simulink model "Actuators"  (Simulink 8.4)
settings: Solver=ode45  StartTime=0.0  StopTime=10.0  RelTol=1e-3
undefined symbols (not defined in the file): Ais_flgAirInjReacPumpOverride, Ais_stAirInjReacPumpMan, Apv_facAirPumpRateMan, Apv_factor, Apv_flgAirPumpRateOverride, Apv_tiPeriod_C, CDRV_E_OK_, Cov_facChOverVlvRateMan, Cov_factor, Cov_flgChOverVlvRateOverride, Cov_tiPeriod_C, Doh_OutputDiagnosisOverride, Fps_flgFuelPumpOverride, Fps_stFuelPumpMan, Icc_degIgnMan, Icc_flgIgnAngleOverride, Icc_flgIgnCutoffMan, Icc_flgIgnCutoffOverride, Icc_nrFollowUpSparks, Icc_tiDwell, Icc_tiDwellFollowUpSparks, Icc_tiOffFollowUpSparks, Ics_flgIntercoolerOverride, Ics_stIntercoolerMan, Ivc_degInjAbort, Ivc_degIntakeClose, Ivc_degOffsetInjEndSimultanInj, Ivc_flgBattDelayOverride, Ivc_flgDiagEntryCondFulfilled, Ivc_flgEndOfStartCond, Ivc_flgInjCutoff, Ivc_flgInjCutoffOverride, Ivc_flgInjTimeOverride, Ivc_flgOverrunCutoff, Ivc_flgPostInjCond, Ivc_tiBattDelayMan, Ivc_tiInjEff, Ivc_tiInjMan, Ivc_tiMinThresDeltaEffInjPeriod, Ivc_weea0, Ivc_weea1, Ivc_weea2, Lo_, Mrs_flgMainRelaisOverride, Mrs_stMainRelaisMan, Normal, OK, OpenCircuit, OverTemp, ShortToBatt, ShortToBattNEG, ShortToGnd, ShortToGndNEG, ShortToGndPOS, Str_flgStarterOverride, Str_stStarterMan, Tvc_facDutycyclePIDLimitMax, Tvc_facDutycyclePIDLimitMin, Tvc_facDutycyclePilotControlNeg, Tvc_facDutycyclePilotControlPos ... (+20)
libraries: simulink x9
(part 1 of 3)
settings Model: Creator=YAL9FE  LastModifiedBy=ric9fe
settings DebuggingCC: FcnCallInpInsideContextMsg=EnableAllAsWarning

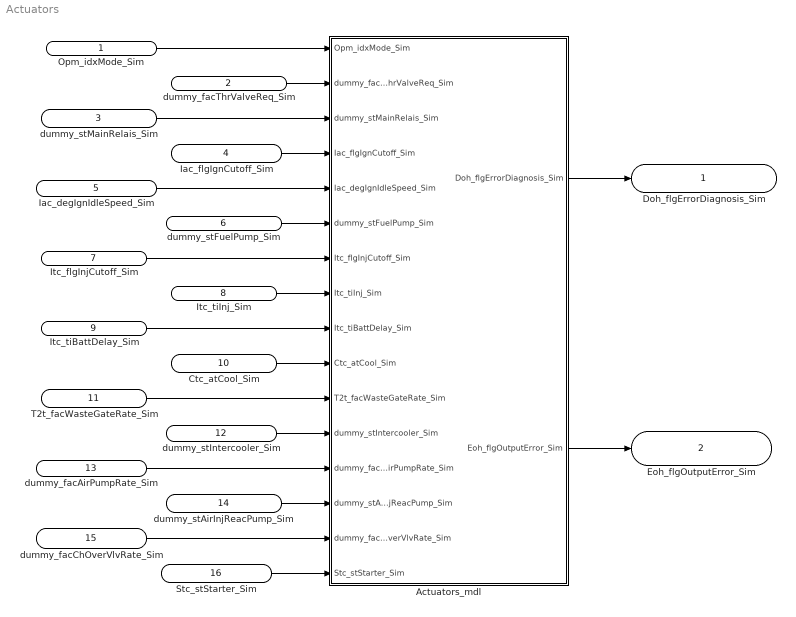
== system Actuators ==
  Opm_idxMode_Sim : Inport
  dummy_facThrValveReq_Sim : Inport  Port=2
  dummy_stMainRelais_Sim : Inport  Port=3
  Iac_flgIgnCutoff_Sim : Inport  Port=4
  Iac_degIgnIdleSpeed_Sim : Inport  Port=5
  dummy_stFuelPump_Sim : Inport  Port=6
  Itc_flgInjCutoff_Sim : Inport  Port=7
  Itc_tiInj_Sim : Inport  Port=8
  Itc_tiBattDelay_Sim : Inport  Port=9
  Ctc_atCool_Sim : Inport  Port=10
  T2t_facWasteGateRate_Sim : Inport  Port=11
  dummy_stIntercooler_Sim : Inport  Port=12
  dummy_facAirPumpRate_Sim : Inport  Port=13
  dummy_stAirInjReacPump_Sim : Inport  Port=14
  dummy_facChOverVlvRate_Sim : Inport  Port=15
  Stc_stStarter_Sim : Inport  Port=16
  Actuators_mdl : Subsystem
  Doh_flgErrorDiagnosis_Sim : Outport
  Eoh_flgOutputError_Sim : Outport  Port=2
  wires:
  Opm_idxMode_Sim/1 -> Actuators_mdl/1(Opm_idxMode_Sim)
  dummy_facThrValveReq_Sim/1 -> Actuators_mdl/2(dummy_facThrValveReq_Sim)
  dummy_stMainRelais_Sim/1 -> Actuators_mdl/3(dummy_stMainRelais_Sim)
  Iac_flgIgnCutoff_Sim/1 -> Actuators_mdl/4(Iac_flgIgnCutoff_Sim)
  Iac_degIgnIdleSpeed_Sim/1 -> Actuators_mdl/5(Iac_degIgnIdleSpeed_Sim)
  dummy_stFuelPump_Sim/1 -> Actuators_mdl/6(dummy_stFuelPump_Sim)
  Itc_flgInjCutoff_Sim/1 -> Actuators_mdl/7(Itc_flgInjCutoff_Sim)
  Itc_tiInj_Sim/1 -> Actuators_mdl/8(Itc_tiInj_Sim)
  Itc_tiBattDelay_Sim/1 -> Actuators_mdl/9(Itc_tiBattDelay_Sim)
  Ctc_atCool_Sim/1 -> Actuators_mdl/10(Ctc_atCool_Sim)
  T2t_facWasteGateRate_Sim/1 -> Actuators_mdl/11(T2t_facWasteGateRate_Sim)
  dummy_stIntercooler_Sim/1 -> Actuators_mdl/12(dummy_stIntercooler_Sim)
  dummy_facAirPumpRate_Sim/1 -> Actuators_mdl/13(dummy_facAirPumpRate_Sim)
  dummy_stAirInjReacPump_Sim/1 -> Actuators_mdl/14(dummy_stAirInjReacPump_Sim)
  dummy_facChOverVlvRate_Sim/1 -> Actuators_mdl/15(dummy_facChOverVlvRate_Sim)
  Stc_stStarter_Sim/1 -> Actuators_mdl/16(Stc_stStarter_Sim)
  Actuators_mdl/1(Doh_flgErrorDiagnosis_Sim) -> Doh_flgErrorDiagnosis_Sim/1
  Actuators_mdl/2(Eoh_flgOutputError_Sim) -> Eoh_flgOutputError_Sim/1

== system Actuators/Actuators_mdl ==
  Opm_idxMode_Sim : Inport
  dummy_facThrValveReq_Sim : Inport  Port=2
  dummy_stMainRelais_Sim : Inport  Port=3
  Iac_flgIgnCutoff_Sim : Inport  Port=4
  Iac_degIgnIdleSpeed_Sim : Inport  Port=5
  dummy_stFuelPump_Sim : Inport  Port=6
  Itc_flgInjCutoff_Sim : Inport  Port=7
  Itc_tiInj_Sim : Inport  Port=8
  Itc_tiBattDelay_Sim : Inport  Port=9
  Ctc_atCool_Sim : Inport  Port=10
  T2t_facWasteGateRate_Sim : Inport  Port=11
  dummy_stIntercooler_Sim : Inport  Port=12
  dummy_facAirPumpRate_Sim : Inport  Port=13
  dummy_stAirInjReacPump_Sim : Inport  Port=14
  dummy_facChOverVlvRate_Sim : Inport  Port=15
  Stc_stStarter_Sim : Inport  Port=16
  Ais : Subsystem  mask(Actuators){}
      mask help: AirInjectionReactorPump
      mask Display:
      | image(imread('AirInjectionReactorPump.jpg'))
      | port_label('input',1,'Opm_idxMode_Sim')
      | port_label('input',2,'dummy_stAirInjReacPump_Sim')
      | port_label('output',1,'Ais_stDiagnosis')
      | port_label('output',2,'Ais_flgError')
  Apv : Subsystem  mask(Actuators){}
      mask help: AirPumpValve
      mask Display:
      | image(imread('AirPumpValve.jpg'))
      | port_label('input',1,'Opm_idxMode_Sim')
      | port_label('input',2,'dummy_facAirPumpRate_Sim')
      | port_label('output',1,'Apv_stDiagnosis')
      | port_label('output',2,'Apv_flgError')
  Cov : Subsystem  mask(Actuators){}
      mask help: ChangeOverValve
      mask Display:
      | image(imread('ChangeOverValve.jpg'))
      | port_label('input',1,'Opm_idxMode_Sim')
      | port_label('input',2,'dummy_facChOverVlvRate_Sim')
      | port_label('output',1,'Cov_stDiagnosis')
      | port_label('output',2,'Cov_flgError')
  Doh : Subsystem  AncestorBlock=M160_lib/Functions/Eih  mask(Functions){}
      mask help: DiagnosisOutput
      mask Display:
      | image(imread('DiagnosisOutput.jpg'))
      | port_label('input',1,'Tvc_stDiagnosis')
      | port_label('input',2,'Mrs_stDiagnosis')
      | port_label('input',3,'Fps_stDiagnosis')
      | port_label('input',4,'Wcs_stDiagnosis')
      | port_label('input',5,'Wgc_stDiagnosis')
      | port_label('input',6,'Ics_stDiagnosis')
      | port_label('input',7,'Apv_stDiagnosis')
      | port_label('input',8,'Ais_stDiagnosis')
      | port_label('input',9,'Cov_stDiagnosis')
      | port_label('input',10,'Str_stDiagnosis')
      | port_label('output',1,'Doh_flgErrorDiagnosis_Sim')
  Eoh : Subsystem  AncestorBlock=M160_lib/Functions/Eih  mask(Functions){}
      mask help: ErrorOutput
      mask Display:
      | image(imread('ErrorOutput.jpg'))
      | port_label('input',1,'Tvc_flgError')
      | port_label('input',2,'Mrs_flgError')
      | port_label('input',3,'Icc_flgError')
      | port_label('input',4,'Fps_flgError')
      | port_label('input',5,'Ivc_flgError')
      | port_label('input',6,'Wcs_flgError')
      | port_label('input',7,'Wgc_flgError')
      | port_label('input',8,'Ics_flgError')
      | port_label('input',9,'Apv_flgError')
      | port_label('input',10,'Ais_flgError')
      | port_label('input',11,'Cov_flgError')
      | port_label('input',12,'Str_flgError')
      | port_label('output',1,'Eoh_flgOutputError_Sim')
  Fps : Subsystem  mask(Actuators){}
      mask help: FuelPump
      mask Display:
      | image(imread('FuelPump.jpg'))
      | port_label('input',1,'Opm_idxMode_Sim')
      | port_label('input',2,'dummy_stFuelPump_Sim')
      | port_label('output',1,'Fps_stDiagnosis')
      | port_label('output',2,'Fps_flgError')
  Icc : Subsystem  mask(Actuators){}
      mask help: IgnitionCoil
      mask Display:
      | image(imread('IgnitionCoil.jpg'))
      | port_label('input',1,'Opm_idxMode_Sim')
      | port_label('input',2,'Iac_flgIgnCutoff_Sim')
      | port_label('input',3,'Iac_degIgnIdleSpeed_Sim')
      | port_label('output',1,'Icc_flgError')
  Ics : Subsystem  mask(Actuators){}
      mask help: Intercooler
      mask Display:
      | image(imread('Intercooler.jpg'))
      | port_label('input',1,'Opm_idxMode_Sim')
      | port_label('input',2,'dummy_stIntercooler_Sim')
      | port_label('output',1,'Ics_stDiagnosis')
      | port_label('output',2,'Ics_flgError')
  Ivc : Subsystem  mask(Actuators){}
      mask help: InjectionValve
      mask Display:
      | image(imread('InjectionValve.jpg'))
      | port_label('input',1,'Opm_idxMode_Sim')
      | port_label('input',2,'Itc_flgInjCutoff_Sim')
      | port_label('input',3,'Itc_tiInj_Sim')
      | port_label('input',4,'Itc_tiBattDelay_Sim')
      | port_label('output',1,'Ivc_flgError')
  Mrs : Subsystem  mask(Actuators){}
      mask help: MainRelais
      mask Display:
      | image(imread('MainRelais.jpg'))
      | port_label('input',1,'Opm_idxMode_Sim')
      | port_label('input',2,'dummy_stMainRelais_Sim')
      | port_label('output',1,'Mrs_stDiagnosis')
      | port_label('output',2,'Mrs_flgError')
  Str : Subsystem  mask(Actuators){}
      mask help: Starter
      mask Display:
      | image(imread('Starter.jpg'))
      | port_label('input',1,'Opm_idxMode_Sim')
      | port_label('input',2,'Stc_stStarter_Sim')
      | port_label('output',1,'Str_stDiagnosis')
      | port_label('output',2,'Str_flgError')
  Tvc : Subsystem  mask(Actuators){}
      mask help: ThrottleValve
      mask Display:
      | image(imread('ThrottleValve.jpg'))
      | port_label('input',1,'Opm_idxMode_Sim')
      | port_label('input',2,'dummy_facThrValveReq_Sim')
      | port_label('output',1,'Tvc_stDiagnosis')
      | port_label('output',2,'Tvc_flgError')
  Wcs : Subsystem  mask(Actuators){}
      mask help: WaterCooler
      mask Display:
      | image(imread('WaterCooler.jpg'))
      | port_label('input',1,'Opm_idxMode_Sim')
      | port_label('input',2,'Ctc_atCool_Sim')
      | port_label('output',1,'Wcs_stDiagnosis')
      | port_label('output',2,'Wcs_flgError')
  Wgc : Subsystem  mask(Actuators){}
      mask help: WasteGate
      mask Display:
      | image(imread('WasteGate.jpg'))
      | port_label('input',1,'Opm_idxMode_Sim')
      | port_label('input',2,'T2t_facWasteGateRate_Sim')
      | port_label('output',1,'Wgc_stDiagnosis')
      | port_label('output',2,'Wgc_flgError')
  Doh_flgErrorDiagnosis_Sim : Outport
  Eoh_flgOutputError_Sim : Outport  Port=2
  wires:
  Icc/1(Icc_flgError) -> Eoh/3(Icc_flgError)
  Mrs/2(Mrs_flgError) -> Eoh/2(Mrs_flgError)
  Tvc/2(Tvc_flgError) -> Eoh/1(Tvc_flgError)
  Eoh/1(Eoh_flgOutputError_Sim) -> Eoh_flgOutputError_Sim/1
  Stc_stStarter_Sim/1 -> Str/2(Stc_stStarter_Sim)
  Str/1(Str_stDiagnosis) -> Doh/10(Str_stDiagnosis)
  dummy_facChOverVlvRate_Sim/1 -> Cov/2(dummy_facChOverVlvRate_Sim)
  Cov/1(Cov_stDiagnosis) -> Doh/9(Cov_stDiagnosis)
  dummy_stAirInjReacPump_Sim/1 -> Ais/2(dummy_stAirInjReacPump_Sim)
  dummy_facAirPumpRate_Sim/1 -> Apv/2(dummy_facAirPumpRate_Sim)
  Fps/2(Fps_flgError) -> Eoh/4(Fps_flgError)
  Ivc/1(Ivc_flgError) -> Eoh/5(Ivc_flgError)
  Wcs/2(Wcs_flgError) -> Eoh/6(Wcs_flgError)
  Wgc/2(Wgc_flgError) -> Eoh/7(Wgc_flgError)
  Ics/2(Ics_flgError) -> Eoh/8(Ics_flgError)
  Apv/2(Apv_flgError) -> Eoh/9(Apv_flgError)
  Ais/2(Ais_flgError) -> Eoh/10(Ais_flgError)
  Cov/2(Cov_flgError) -> Eoh/11(Cov_flgError)
  Str/2(Str_flgError) -> Eoh/12(Str_flgError)
  Doh/1(Doh_flgErrorDiagnosis_Sim) -> Doh_flgErrorDiagnosis_Sim/1
  Opm_idxMode_Sim/1 -> Tvc/1(Opm_idxMode_Sim), Mrs/1(Opm_idxMode_Sim), Icc/1(Opm_idxMode_Sim), Fps/1(Opm_idxMode_Sim), Ivc/1(Opm_idxMode_Sim), Wcs/1(Opm_idxMode_Sim), Wgc/1(Opm_idxMode_Sim), Apv/1(Opm_idxMode_Sim), Ais/1(Opm_idxMode_Sim), Cov/1(Opm_idxMode_Sim), Str/1(Opm_idxMode_Sim), Ics/1(Opm_idxMode_Sim)
  Ais/1(Ais_stDiagnosis) -> Doh/8(Ais_stDiagnosis)
  Apv/1(Apv_stDiagnosis) -> Doh/7(Apv_stDiagnosis)
  dummy_stIntercooler_Sim/1 -> Ics/2(dummy_stIntercooler_Sim)
  Ics/1(Ics_stDiagnosis) -> Doh/6(Ics_stDiagnosis)
  T2t_facWasteGateRate_Sim/1 -> Wgc/2(T2t_facWasteGateRate_Sim)
  Wgc/1(Wgc_stDiagnosis) -> Doh/5(Wgc_stDiagnosis)
  Ctc_atCool_Sim/1 -> Wcs/2(Ctc_atCool_Sim)
  Wcs/1(Wcs_stDiagnosis) -> Doh/4(Wcs_stDiagnosis)
  Itc_tiBattDelay_Sim/1 -> Ivc/4(Itc_tiBattDelay_Sim)
  Itc_tiInj_Sim/1 -> Ivc/3(Itc_tiInj_Sim)
  Itc_flgInjCutoff_Sim/1 -> Ivc/2(Itc_flgInjCutoff_Sim)
  dummy_stFuelPump_Sim/1 -> Fps/2(dummy_stFuelPump_Sim)
  Fps/1(Fps_stDiagnosis) -> Doh/3(Fps_stDiagnosis)
  Iac_degIgnIdleSpeed_Sim/1 -> Icc/3(Iac_degIgnIdleSpeed_Sim)
  Iac_flgIgnCutoff_Sim/1 -> Icc/2(Iac_flgIgnCutoff_Sim)
  dummy_stMainRelais_Sim/1 -> Mrs/2(dummy_stMainRelais_Sim)
  Mrs/1(Mrs_stDiagnosis) -> Doh/2(Mrs_stDiagnosis)
  Tvc/1(Tvc_stDiagnosis) -> Doh/1(Tvc_stDiagnosis)
  dummy_facThrValveReq_Sim/1 -> Tvc/2(dummy_facThrValveReq_Sim)
  ? -> Cov/Trigger

== system Actuators/Actuators_mdl/Ais ==
  Opm_idxMode_Sim : Inport
  dummy_stAirInjReacPump_Sim : Inport  Port=2
  function : TriggerPort  TriggerType=function-call
  Constant1 : Constant  Value=Ais_flgAirInjReacPumpOverride
  Constant2 : Constant  Value=Ais_stAirInjReacPumpMan
  Constant5 : Constant  Value=Normal
  Constant6 : Constant  Value=0  OutDataTypeStr=boolean
  G1_DigOut_Ctrl : Subsystem  AncestorBlock=ehooks_medc17flex_G1_lib/Library Blocks/Basic_IO/Outputs/G1_DigOut_Ctrl  mask{ChannelName=O_S_RL30}
      mask prompts: ChannelName "Channel name"
      mask init:
      | ehooks_medc17flex_devlib_io_block('mask_init');
      settings: AttributesFormatString=Channel name: '%<ChannelName>'
      mask TypeOptions ChannelName: <empty> | O_S_MRLY | O_S_RL09 | O_S_RL14 | O_S_RL29 | O_S_RL30 | O_S_RL31 | O_S_RL33 | O_S_RL34 | O_S_RL35 | O_S_RL41 | O_S_RL43
      mask Display: image(imread('Output_Digital.jpg'))
  G1_DigOut_GetError : Subsystem  AncestorBlock=ehooks_medc17flex_G1_lib/Library Blocks/Basic_IO/Outputs/G1_DigOut_GetError  mask{ChannelName=O_S_RL30}
      mask prompts: ChannelName "Channel name"
      mask init:
      | ehooks_medc17flex_devlib_io_block('mask_init');
      settings: AttributesFormatString=Channel name: '%<ChannelName>'
      mask TypeOptions ChannelName: <empty> | O_S_MRLY | O_S_RL09 | O_S_RL14 | O_S_RL29 | O_S_RL30 | O_S_RL31 | O_S_RL33 | O_S_RL34 | O_S_RL35 | O_S_RL41 | O_S_RL43
      mask Display: image(imread('Output_Digital_Diagnosis.jpg'))
  Logical Operator1 : Logic  Operator=NOT  AllPortsSameDT=off  OutDataTypeStr=boolean
  Logical Operator2 : Logic  Operator=NOT  AllPortsSameDT=off  OutDataTypeStr=boolean
  Relational Operator : RelationalOperator  Operator===  OutDataTypeStr=boolean
  Switch1 : Switch  Threshold=1
  Switch2 : Switch  Threshold=1
  Ais_stDiagnosis : Outport
  Ais_flgError : Outport  Port=2
  wires:
  G1_DigOut_Ctrl/1(status) -> Logical Operator1/1
  Logical Operator2/1 -> G1_DigOut_Ctrl/1(state)
  Switch2/1 -> Logical Operator2/1  "Ais_stAirInjReacPump"
  G1_DigOut_GetError/1(status) -> Ais_stDiagnosis/1  "Ais_stDiagnosis"
  Logical Operator1/1 -> Ais_flgError/1  "Ais_flgError"
  Constant1/1 -> Switch1/2
  Constant2/1 -> Switch1/1
  dummy_stAirInjReacPump_Sim/1 -> Switch1/3
  Switch1/1 -> Switch2/1
  Opm_idxMode_Sim/1 -> Relational Operator/1
  Constant5/1 -> Relational Operator/2
  Relational Operator/1 -> Switch2/2
  Constant6/1 -> Switch2/3

== system Actuators/Actuators_mdl/Apv ==
  Opm_idxMode_Sim : Inport
  dummy_facAirPumpRate_Sim : Inport  Port=2
  function : TriggerPort  TriggerType=function-call
  Constant1 : Constant  Value=Apv_flgAirPumpRateOverride
  Constant2 : Constant  Value=Apv_facAirPumpRateMan
  Constant3 : Constant  Value=10000  OutDataTypeStr=single
  Constant4 : Constant  Value=Apv_factor
  Constant5 : Constant  Value=Normal
  Constant6 : Constant  Value=0.05  OutDataTypeStr=single
  Constant7 : Constant  Value=Apv_tiPeriod_C
  Constant9 : Constant  Value=Lo_
  G1_PWM_Output_Ctrl : Subsystem  AncestorBlock=ehooks_medc17flex_G1_lib/Library Blocks/Basic_IO/Outputs/G1_PWM_Output_Ctrl  mask{ChannelName=O_T_RL13}
      mask prompts: ChannelName "Channel name"
      mask init:
      | ehooks_medc17flex_devlib_io_block('mask_init');
      settings: AttributesFormatString=Channel name: '%<ChannelName>'
      mask TypeOptions ChannelName: <empty> | O_T_RL10 | O_T_RL13 | O_T_RL19 | O_T_RL20 | O_T_RL22 | O_T_RL23 | O_T_RL25 | O_T_RL26 | O_T_RL27 | O_T_RL28 | O_T_RL38 | O_T_RL39 | O_T_RL40 | O_T_RL42 | O_T_RL44 | O_T_RL45 | O_T_RL46 | O_T_RL47 | O_T_RL48 | O_T_RL49 | O_T_RL50 | O_T_RH02
      mask Display: image(imread('Output_PWM.jpg'))
  G1_PwmOut_Get_error : Subsystem  AncestorBlock=ehooks_medc17flex_G1_lib/Library Blocks/Basic_IO/Outputs/G1_PwmOut_Get_error  mask{ChannelName=O_T_RL13}
      mask prompts: ChannelName "Channel name"
      mask init:
      | ehooks_medc17flex_devlib_io_block('mask_init');
      settings: AttributesFormatString=Channel name: '%<ChannelName>'
      mask TypeOptions ChannelName: <empty> | O_T_RL10 | O_T_RL13 | O_T_RL19 | O_T_RL20 | O_T_RL22 | O_T_RL23 | O_T_RL25 | O_T_RL26 | O_T_RL27 | O_T_RL28 | O_T_RL38 | O_T_RL39 | O_T_RL40 | O_T_RL42 | O_T_RL44 | O_T_RL45 | O_T_RL46 | O_T_RL47 | O_T_RL48 | O_T_RL49 | O_T_RL50 | O_T_RH02
      mask Display: image(imread('Output_PWM_Diagnosis.jpg'))
  Logical Operator1 : Logic  Operator=NOT  AllPortsSameDT=off  OutDataTypeStr=boolean
  Product1 : Product  OutDataTypeStr=Inherit: Same as first input
  Relational Operator : RelationalOperator  Operator===  OutDataTypeStr=boolean
  Switch1 : Switch  Threshold=1
  Switch2 : Switch  Threshold=1
  Apv_stDiagnosis : Outport
  Apv_flgError : Outport  Port=2
  wires:
  Constant9/1 -> G1_PWM_Output_Ctrl/4(level)
  Constant4/1 -> G1_PWM_Output_Ctrl/3(factor)
  Constant7/1 -> G1_PWM_Output_Ctrl/2(period)
  Product1/1 -> G1_PWM_Output_Ctrl/1(dutycycle)
  Constant3/1 -> Product1/2
  G1_PWM_Output_Ctrl/1(status) -> Logical Operator1/1
  Switch2/1 -> Product1/1  "Apv_facAirPumpRate"
  G1_PwmOut_Get_error/1(status) -> Apv_stDiagnosis/1  "Apv_stDiagnosis"
  Logical Operator1/1 -> Apv_flgError/1  "Apv_flgError"
  Constant1/1 -> Switch1/2
  Constant2/1 -> Switch1/1
  dummy_facAirPumpRate_Sim/1 -> Switch1/3
  Switch1/1 -> Switch2/1
  Opm_idxMode_Sim/1 -> Relational Operator/1
  Constant5/1 -> Relational Operator/2
  Relational Operator/1 -> Switch2/2
  Constant6/1 -> Switch2/3

== system Actuators/Actuators_mdl/Cov ==
  Opm_idxMode_Sim : Inport
  dummy_facChOverVlvRate_Sim : Inport  Port=2
  function : TriggerPort  TriggerType=function-call
  Constant1 : Constant  Value=Cov_flgChOverVlvRateOverride
  Constant2 : Constant  Value=Cov_facChOverVlvRateMan
  Constant3 : Constant  Value=10000  OutDataTypeStr=single
  Constant4 : Constant  Value=Cov_factor
  Constant5 : Constant  Value=Normal
  Constant6 : Constant  Value=0.05  OutDataTypeStr=single
  Constant7 : Constant  Value=Cov_tiPeriod_C
  Constant9 : Constant  Value=Lo_
  G1_PWM_Output_Ctrl : Subsystem  AncestorBlock=ehooks_medc17flex_G1_lib/Library Blocks/Basic_IO/Outputs/G1_PWM_Output_Ctrl  mask{ChannelName=O_T_RL10}
      mask prompts: ChannelName "Channel name"
      mask init:
      | ehooks_medc17flex_devlib_io_block('mask_init');
      settings: AttributesFormatString=Channel name: '%<ChannelName>'
      mask TypeOptions ChannelName: <empty> | O_T_RL10 | O_T_RL13 | O_T_RL19 | O_T_RL20 | O_T_RL22 | O_T_RL23 | O_T_RL25 | O_T_RL26 | O_T_RL27 | O_T_RL28 | O_T_RL38 | O_T_RL39 | O_T_RL40 | O_T_RL42 | O_T_RL44 | O_T_RL45 | O_T_RL46 | O_T_RL47 | O_T_RL48 | O_T_RL49 | O_T_RL50 | O_T_RH02
      mask Display: image(imread('Output_PWM.jpg'))
  G1_PwmOut_Get_error : Subsystem  AncestorBlock=ehooks_medc17flex_G1_lib/Library Blocks/Basic_IO/Outputs/G1_PwmOut_Get_error  mask{ChannelName=O_T_RL10}
      mask prompts: ChannelName "Channel name"
      mask init:
      | ehooks_medc17flex_devlib_io_block('mask_init');
      settings: AttributesFormatString=Channel name: '%<ChannelName>'
      mask TypeOptions ChannelName: <empty> | O_T_RL10 | O_T_RL13 | O_T_RL19 | O_T_RL20 | O_T_RL22 | O_T_RL23 | O_T_RL25 | O_T_RL26 | O_T_RL27 | O_T_RL28 | O_T_RL38 | O_T_RL39 | O_T_RL40 | O_T_RL42 | O_T_RL44 | O_T_RL45 | O_T_RL46 | O_T_RL47 | O_T_RL48 | O_T_RL49 | O_T_RL50 | O_T_RH02
      mask Display: image(imread('Output_PWM_Diagnosis.jpg'))
  Logical Operator1 : Logic  Operator=NOT  AllPortsSameDT=off  OutDataTypeStr=boolean
  Product1 : Product  OutDataTypeStr=Inherit: Same as first input
  Relational Operator : RelationalOperator  Operator===  OutDataTypeStr=boolean
  Switch1 : Switch  Threshold=1
  Switch2 : Switch  Threshold=1
  Cov_stDiagnosis : Outport
  Cov_flgError : Outport  Port=2
  wires:
  Constant6/1 -> Switch2/3
  Relational Operator/1 -> Switch2/2
  Constant5/1 -> Relational Operator/2
  Opm_idxMode_Sim/1 -> Relational Operator/1
  Switch1/1 -> Switch2/1
  dummy_facChOverVlvRate_Sim/1 -> Switch1/3
  Constant2/1 -> Switch1/1
  Constant1/1 -> Switch1/2
  Logical Operator1/1 -> Cov_flgError/1  "Cov_flgError"
  G1_PwmOut_Get_error/1(status) -> Cov_stDiagnosis/1  "Cov_stDiagnosis"
  Switch2/1 -> Product1/1  "Cov_facChOverVlvRate"
  G1_PWM_Output_Ctrl/1(status) -> Logical Operator1/1
  Constant3/1 -> Product1/2
  Product1/1 -> G1_PWM_Output_Ctrl/1(dutycycle)
  Constant7/1 -> G1_PWM_Output_Ctrl/2(period)
  Constant4/1 -> G1_PWM_Output_Ctrl/3(factor)
  Constant9/1 -> G1_PWM_Output_Ctrl/4(level)

== system Actuators/Actuators_mdl/Doh ==
  Tvc_stDiagnosis : Inport
  Mrs_stDiagnosis : Inport  Port=2
  Fps_stDiagnosis : Inport  Port=3
  Wcs_stDiagnosis : Inport  Port=4
  Wgc_stDiagnosis : Inport  Port=5
  Ics_stDiagnosis : Inport  Port=6
  Apv_stDiagnosis : Inport  Port=7
  Ais_stDiagnosis : Inport  Port=8
  Cov_stDiagnosis : Inport  Port=9
  Str_stDiagnosis : Inport  Port=10
  function : TriggerPort  TriggerType=function-call
  Constant1 : Constant  Value=Doh_OutputDiagnosisOverride
  Constant6 : Constant  Value=0  OutDataTypeStr=boolean
  DiagnosisOutput_1 : Subsystem
  DiagnosisOutput_10 : Subsystem
  DiagnosisOutput_2 : Subsystem
  DiagnosisOutput_3 : Subsystem
  DiagnosisOutput_4 : Subsystem
  DiagnosisOutput_5 : Subsystem
  DiagnosisOutput_6 : Subsystem
  DiagnosisOutput_7 : Subsystem
  DiagnosisOutput_8 : Subsystem
  DiagnosisOutput_9 : Subsystem
  Logical Operator4 : Logic  Operator=OR  Inputs=10  AllPortsSameDT=off  OutDataTypeStr=boolean
  Switch2 : Switch  Threshold=1
  Doh_flgErrorDiagnosis_Sim : Outport
  wires:
  Constant1/1 -> Switch2/2
  Switch2/1 -> Doh_flgErrorDiagnosis_Sim/1  "Doh_flgErrorDiagnosis_Sim"
  Constant6/1 -> Switch2/1
  Logical Operator4/1 -> Switch2/3
  Tvc_stDiagnosis/1 -> DiagnosisOutput_1/1(status)
  DiagnosisOutput_1/1(stError) -> Logical Operator4/1
  Mrs_stDiagnosis/1 -> DiagnosisOutput_2/1(status)
  DiagnosisOutput_2/1(stError) -> Logical Operator4/2
  Fps_stDiagnosis/1 -> DiagnosisOutput_3/1(status)
  DiagnosisOutput_3/1(stError) -> Logical Operator4/3
  Wcs_stDiagnosis/1 -> DiagnosisOutput_4/1(status)
  DiagnosisOutput_4/1(stError) -> Logical Operator4/4
  Wgc_stDiagnosis/1 -> DiagnosisOutput_5/1(status)
  DiagnosisOutput_5/1(stError) -> Logical Operator4/5
  Ics_stDiagnosis/1 -> DiagnosisOutput_6/1(status)
  DiagnosisOutput_6/1(stError) -> Logical Operator4/6
  Apv_stDiagnosis/1 -> DiagnosisOutput_7/1(status)
  DiagnosisOutput_7/1(stError) -> Logical Operator4/7
  Ais_stDiagnosis/1 -> DiagnosisOutput_8/1(status)
  DiagnosisOutput_8/1(stError) -> Logical Operator4/8
  Cov_stDiagnosis/1 -> DiagnosisOutput_9/1(status)
  DiagnosisOutput_9/1(stError) -> Logical Operator4/9
  Str_stDiagnosis/1 -> DiagnosisOutput_10/1(status)
  DiagnosisOutput_10/1(stError) -> Logical Operator4/10

== system Actuators/Actuators_mdl/Eoh ==
  Tvc_flgError : Inport
  Mrs_flgError : Inport  Port=2
  Icc_flgError : Inport  Port=3
  Fps_flgError : Inport  Port=4
  Ivc_flgError : Inport  Port=5
  Wcs_flgError : Inport  Port=6
  Wgc_flgError : Inport  Port=7
  Ics_flgError : Inport  Port=8
  Apv_flgError : Inport  Port=9
  Ais_flgError : Inport  Port=10
  Cov_flgError : Inport  Port=11
  Str_flgError : Inport  Port=12
  function : TriggerPort  TriggerType=function-call
  Logical Operator4 : Logic  Operator=OR  Inputs=12  AllPortsSameDT=off  OutDataTypeStr=boolean
  Eoh_flgOutputError_Sim : Outport
  wires:
  Logical Operator4/1 -> Eoh_flgOutputError_Sim/1  "Eoh_flgOutputError_Sim"
  Tvc_flgError/1 -> Logical Operator4/1
  Mrs_flgError/1 -> Logical Operator4/2
  Icc_flgError/1 -> Logical Operator4/3
  Fps_flgError/1 -> Logical Operator4/4
  Ivc_flgError/1 -> Logical Operator4/5
  Wcs_flgError/1 -> Logical Operator4/6
  Wgc_flgError/1 -> Logical Operator4/7
  Ics_flgError/1 -> Logical Operator4/8
  Apv_flgError/1 -> Logical Operator4/9
  Ais_flgError/1 -> Logical Operator4/10
  Cov_flgError/1 -> Logical Operator4/11
  Str_flgError/1 -> Logical Operator4/12

== system Actuators/Actuators_mdl/Fps ==
  Opm_idxMode_Sim : Inport
  dummy_stFuelPump_Sim : Inport  Port=2
  function : TriggerPort  TriggerType=function-call
  Constant1 : Constant  Value=Fps_flgFuelPumpOverride
  Constant2 : Constant  Value=Fps_stFuelPumpMan
  Constant5 : Constant  Value=Normal
  Constant6 : Constant  Value=0  OutDataTypeStr=boolean
  G1_DigOut_Ctrl : Subsystem  AncestorBlock=ehooks_medc17flex_G1_lib/Library Blocks/Basic_IO/Outputs/G1_DigOut_Ctrl  mask{ChannelName=O_S_RL09}
      mask prompts: ChannelName "Channel name"
      mask init:
      | ehooks_medc17flex_devlib_io_block('mask_init');
      settings: AttributesFormatString=Channel name: '%<ChannelName>'
      mask TypeOptions ChannelName: <empty> | O_S_MRLY | O_S_RL09 | O_S_RL14 | O_S_RL29 | O_S_RL30 | O_S_RL31 | O_S_RL33 | O_S_RL34 | O_S_RL35 | O_S_RL41 | O_S_RL43
      mask Display: image(imread('Output_Digital.jpg'))
  G1_DigOut_GetError : Subsystem  AncestorBlock=ehooks_medc17flex_G1_lib/Library Blocks/Basic_IO/Outputs/G1_DigOut_GetError  mask{ChannelName=O_S_RL09}
      mask prompts: ChannelName "Channel name"
      mask init:
      | ehooks_medc17flex_devlib_io_block('mask_init');
      settings: AttributesFormatString=Channel name: '%<ChannelName>'
      mask TypeOptions ChannelName: <empty> | O_S_MRLY | O_S_RL09 | O_S_RL14 | O_S_RL29 | O_S_RL30 | O_S_RL31 | O_S_RL33 | O_S_RL34 | O_S_RL35 | O_S_RL41 | O_S_RL43
      mask Display: image(imread('Output_Digital_Diagnosis.jpg'))
  Logical Operator1 : Logic  Operator=NOT  AllPortsSameDT=off  OutDataTypeStr=boolean
  Logical Operator2 : Logic  Operator=NOT  AllPortsSameDT=off  OutDataTypeStr=boolean
  Relational Operator : RelationalOperator  Operator===  OutDataTypeStr=boolean
  Switch1 : Switch  Threshold=1
  Switch2 : Switch  Threshold=1
  Fps_stDiagnosis : Outport
  Fps_flgError : Outport  Port=2
  wires:
  G1_DigOut_Ctrl/1(status) -> Logical Operator1/1
  Logical Operator2/1 -> G1_DigOut_Ctrl/1(state)
  Switch2/1 -> Logical Operator2/1  "Fps_stFuelPump"
  G1_DigOut_GetError/1(status) -> Fps_stDiagnosis/1  "Fps_stDiagnosis"
  Logical Operator1/1 -> Fps_flgError/1  "Fps_flgError"
  Constant1/1 -> Switch1/2
  Constant2/1 -> Switch1/1
  dummy_stFuelPump_Sim/1 -> Switch1/3
  Switch1/1 -> Switch2/1
  Opm_idxMode_Sim/1 -> Relational Operator/1
  Constant5/1 -> Relational Operator/2
  Relational Operator/1 -> Switch2/2
  Constant6/1 -> Switch2/3

== system Actuators/Actuators_mdl/Icc ==
  note: PlaceHolder
  note: PlaceHolder
  Opm_idxMode_Sim : Inport
  Iac_flgIgnCutoff_Sim : Inport  Port=2
  Iac_degIgnIdleSpeed_Sim : Inport  Port=3
  function : TriggerPort  TriggerType=function-call
  Constant1 : Constant  Value=Icc_flgIgnCutoffOverride
  Constant10 : Constant  Value=Icc_tiOffFollowUpSparks
  Constant11 : Constant  Value=Icc_nrFollowUpSparks
  Constant{6,12..15} (5 alike) : Constant  Value=0  OutMin=-72  OutMax=78  OutDataTypeStr=single
  Constant2 : Constant  Value=Icc_flgIgnCutoffMan
  Constant3 : Constant  Value=CDRV_E_OK_
  Constant4 : Constant  Value=Icc_flgIgnAngleOverride
  Constant5 : Constant  Value=Normal
  Constant7 : Constant  Value=Icc_degIgnMan
  Constant8 : Constant  Value=Icc_tiDwell
  Constant9 : Constant  Value=Icc_tiDwellFollowUpSparks
  Demux : Demux  Outputs=8
  EdgeFalling : Subsystem
      mask help: EdgeFalling
      mask Display: image(imread('EdgeFalling.jpg'))
  EdgeRising : Subsystem
      mask help: EdgeRising
      mask Display: image(imread('EdgeRising.jpg'))
  G1_IGN_SetParam_for_PFI : Subsystem  AncestorBlock=ehooks_medc17flex_G1_lib/Library Blocks/IGN/IGN_PFI_Specific/G1_IGN_SetParam_for_PFI  mask{handleName=IGNORED}
      mask prompts: handleName "PlaceHolder_IGNORED"
      mask init:
      | ehooks_medc17flex_devlib_io_block('mask_init');
      mask TypeOptions handleName: IGNORED
      mask Display: image(imread('IgnClPfi.jpg'))
  IGN_FadeOut_Immediate : Subsystem  Priority=44  AncestorBlock=ehooks_medc17flex_G1_lib/Library Blocks/IGN/IGN_Fadeout/IGN_FadeOut_Immediate  mask{ChannelName=IGNORED}
      mask prompts: ChannelName "PlaceHolder_IGNORED"
      mask init:
      | ehooks_medc17flex_devlib_io_block('mask_init');
      mask TypeOptions ChannelName: IGNORED
  Logical Operator3 : Logic  Operator=OR  AllPortsSameDT=off  OutDataTypeStr=boolean
  Relational Operator : RelationalOperator  Operator=~=  OutDataTypeStr=boolean
  Relational Operator1 : RelationalOperator  Operator=~=  OutDataTypeStr=boolean
  Switch1 : Switch  Threshold=1
  Switch2 : Switch  Threshold=1
  Vector Concatenate : Concatenate  NumInputs=8
  fadeIn : Terminator
  fadeOut : Terminator
  Icc_flgError : Outport
  wires:
  Constant1/1 -> Switch1/2
  Constant2/1 -> Switch1/1
  Iac_flgIgnCutoff_Sim/1 -> Switch1/3
  Opm_idxMode_Sim/1 -> Relational Operator/1
  Constant5/1 -> Relational Operator/2
  G1_IGN_SetParam_for_PFI/1(status) -> Relational Operator1/1  "Icc_idxPfiCdrvInterfaceError"
  Relational Operator1/1 -> Icc_flgError/1  "Icc_flgError"
  Constant3/1 -> Relational Operator1/2
  Iac_degIgnIdleSpeed_Sim/1 -> Switch2/3
  Constant4/1 -> Switch2/2
  Constant7/1 -> Switch2/1
  Relational Operator/1 -> Logical Operator3/1
  Switch1/1 -> Logical Operator3/2
  Constant8/1 -> G1_IGN_SetParam_for_PFI/1(szout_w)
  Constant9/1 -> G1_IGN_SetParam_for_PFI/2(szfuba_w)
  Constant10/1 -> G1_IGN_SetParam_for_PFI/3(offz_w)
  Constant11/1 -> G1_IGN_SetParam_for_PFI/12(IGN_fubaanz)
  Logical Operator3/1 -> EdgeRising/1(signal), EdgeFalling/1(signal)  "Icc_stIgnFadeOutReq"
  Demux/1 -> G1_IGN_SetParam_for_PFI/4(IGN_zwcalcar_1)
  Demux/2 -> G1_IGN_SetParam_for_PFI/5(IGN_zwcalcar_2)
  Demux/3 -> G1_IGN_SetParam_for_PFI/6(IGN_zwcalcar_3)
  Demux/4 -> G1_IGN_SetParam_for_PFI/7(IGN_zwcalcar_4)
  Demux/5 -> G1_IGN_SetParam_for_PFI/8(IGN_zwcalcar_5)
  Demux/6 -> G1_IGN_SetParam_for_PFI/9(IGN_zwcalcar_6)
  Demux/7 -> G1_IGN_SetParam_for_PFI/10(IGN_zwcalcar_7)
  Demux/8 -> G1_IGN_SetParam_for_PFI/11(IGN_zwcalcar_8)
  Vector Concatenate/1 -> Demux/1  "Icc_degIgn_Arr"
  Constant6/1 -> Vector Concatenate/4
  Constant12/1 -> Vector Concatenate/5
  Constant13/1 -> Vector Concatenate/6
  Constant14/1 -> Vector Concatenate/7
  Constant15/1 -> Vector Concatenate/8
  Switch2/1 -> Vector Concatenate/1, Vector Concatenate/3, Vector Concatenate/2
  EdgeFalling/1(return) -> fadeIn/1
  EdgeRising/1(return) -> fadeOut/1

== system Actuators/Actuators_mdl/Ics ==
  Opm_idxMode_Sim : Inport
  dummy_stIntercooler_Sim : Inport  Port=2
  function : TriggerPort  TriggerType=function-call
  Constant1 : Constant  Value=Ics_flgIntercoolerOverride
  Constant2 : Constant  Value=Ics_stIntercoolerMan
  Constant5 : Constant  Value=Normal
  Constant6 : Constant  Value=0  OutDataTypeStr=boolean
  G1_DigOut_Ctrl : Subsystem  AncestorBlock=ehooks_medc17flex_G1_lib/Library Blocks/Basic_IO/Outputs/G1_DigOut_Ctrl  mask{ChannelName=O_S_RL29}
      mask prompts: ChannelName "Channel name"
      mask init:
      | ehooks_medc17flex_devlib_io_block('mask_init');
      settings: AttributesFormatString=Channel name: '%<ChannelName>'
      mask TypeOptions ChannelName: <empty> | O_S_MRLY | O_S_RL09 | O_S_RL14 | O_S_RL29 | O_S_RL30 | O_S_RL31 | O_S_RL33 | O_S_RL34 | O_S_RL35 | O_S_RL41 | O_S_RL43
      mask Display: image(imread('Output_Digital.jpg'))
  G1_DigOut_GetError : Subsystem  AncestorBlock=ehooks_medc17flex_G1_lib/Library Blocks/Basic_IO/Outputs/G1_DigOut_GetError  mask{ChannelName=O_S_RL29}
      mask prompts: ChannelName "Channel name"
      mask init:
      | ehooks_medc17flex_devlib_io_block('mask_init');
      settings: AttributesFormatString=Channel name: '%<ChannelName>'
      mask TypeOptions ChannelName: <empty> | O_S_MRLY | O_S_RL09 | O_S_RL14 | O_S_RL29 | O_S_RL30 | O_S_RL31 | O_S_RL33 | O_S_RL34 | O_S_RL35 | O_S_RL41 | O_S_RL43
      mask Display: image(imread('Output_Digital_Diagnosis.jpg'))
  Logical Operator1 : Logic  Operator=NOT  AllPortsSameDT=off  OutDataTypeStr=boolean
  Logical Operator2 : Logic  Operator=NOT  AllPortsSameDT=off  OutDataTypeStr=boolean
  Relational Operator : RelationalOperator  Operator===  OutDataTypeStr=boolean
  Switch1 : Switch  Threshold=1
  Switch2 : Switch  Threshold=1
  Ics_stDiagnosis : Outport
  Ics_flgError : Outport  Port=2
  wires:
  Constant6/1 -> Switch2/3
  Relational Operator/1 -> Switch2/2
  Constant5/1 -> Relational Operator/2
  Opm_idxMode_Sim/1 -> Relational Operator/1
  Switch1/1 -> Switch2/1
  dummy_stIntercooler_Sim/1 -> Switch1/3
  Constant2/1 -> Switch1/1
  Constant1/1 -> Switch1/2
  Logical Operator1/1 -> Ics_flgError/1  "Ics_flgError"
  G1_DigOut_GetError/1(status) -> Ics_stDiagnosis/1  "Ics_stDiagnosis"
  Switch2/1 -> Logical Operator2/1  "Ics_stIntercooler"
  Logical Operator2/1 -> G1_DigOut_Ctrl/1(state)
  G1_DigOut_Ctrl/1(status) -> Logical Operator1/1

== system Actuators/Actuators_mdl/Ivc ==
  Opm_idxMode_Sim : Inport
  Itc_flgInjCutoff_Sim : Inport  Port=2
  Itc_tiInj_Sim : Inport  Port=3
  Itc_tiBattDelay_Sim : Inport  Port=4
  Ivc : Subsystem  mask(Actuators){}
      mask help: InjectionValve
      mask Display:
      | image(imread('InjectionValve.jpg'))
      | port_label('input',1,'Opm_idxMode_Sim')
      | port_label('input',2,'Itc_flgInjCutoff_Sim')
      | port_label('input',3,'Itc_tiInj_Sim')
      | port_label('input',4,'Itc_tiBattDelay_Sim')
      | port_label('output',1,'Ivc_flgError')
  Ivc_Diag : Subsystem  mask(Actuators){}
      mask help: InjectionValveDiagnose
      mask Display:
      | image(imread('InjectionValve.jpg'))
      | port_label('output',1,'Ivc_flgError')
  Ivc_Error : Subsystem  mask(Actuators){}
      mask help: InjectionValveError
      mask Display:
      | image(imread('InjectionValve.jpg'))
      | port_label('output',1,'Ivc_flgError')
  Ivc_flgError : Outport
  wires:
  Opm_idxMode_Sim/1 -> Ivc/1(Opm_idxMode_Sim)
  Itc_flgInjCutoff_Sim/1 -> Ivc/2(Itc_flgInjCutoff_Sim)
  Itc_tiInj_Sim/1 -> Ivc/3(Itc_tiInj_Sim)
  Itc_tiBattDelay_Sim/1 -> Ivc/4(Itc_tiBattDelay_Sim)
  Ivc/1(Ivc_flgError) -> Ivc_Error/1(Ivc)
  Ivc_Diag/1(Ivc_flgError) -> Ivc_Error/2(Ivc_Diag)
  Ivc_Error/1(Ivc_flgError) -> Ivc_flgError/1

== system Actuators/Actuators_mdl/Mrs ==
  Opm_idxMode_Sim : Inport
  dummy_stMainRelais_Sim : Inport  Port=2
  function : TriggerPort  TriggerType=function-call
  Constant1 : Constant  Value=Mrs_flgMainRelaisOverride
  Constant2 : Constant  Value=Mrs_stMainRelaisMan
  Constant5 : Constant  Value=Normal
  Constant6 : Constant  OutDataTypeStr=boolean
  G1_DigOut_Ctrl : Subsystem  AncestorBlock=ehooks_medc17flex_G1_lib/Library Blocks/Basic_IO/Outputs/G1_DigOut_Ctrl  mask{ChannelName=O_S_MRLY}
      mask prompts: ChannelName "Channel name"
      mask init:
      | ehooks_medc17flex_devlib_io_block('mask_init');
      settings: AttributesFormatString=Channel name: '%<ChannelName>'
      mask TypeOptions ChannelName: <empty> | O_S_MRLY | O_S_RL09 | O_S_RL14 | O_S_RL29 | O_S_RL30 | O_S_RL31 | O_S_RL33 | O_S_RL34 | O_S_RL35 | O_S_RL41 | O_S_RL43
      mask Display: image(imread('Output_Digital.jpg'))
  G1_DigOut_GetError : Subsystem  AncestorBlock=ehooks_medc17flex_G1_lib/Library Blocks/Basic_IO/Outputs/G1_DigOut_GetError  mask{ChannelName=O_S_MRLY}
      mask prompts: ChannelName "Channel name"
      mask init:
      | ehooks_medc17flex_devlib_io_block('mask_init');
      settings: AttributesFormatString=Channel name: '%<ChannelName>'
      mask TypeOptions ChannelName: <empty> | O_S_MRLY | O_S_RL09 | O_S_RL14 | O_S_RL29 | O_S_RL30 | O_S_RL31 | O_S_RL33 | O_S_RL34 | O_S_RL35 | O_S_RL41 | O_S_RL43
      mask Display: image(imread('Output_Digital_Diagnosis.jpg'))
  Logical Operator1 : Logic  Operator=NOT  AllPortsSameDT=off  OutDataTypeStr=boolean
  Logical Operator2 : Logic  Operator=NOT  AllPortsSameDT=off  OutDataTypeStr=boolean
  Relational Operator : RelationalOperator  Operator===  OutDataTypeStr=boolean
  Switch1 : Switch  Threshold=1
  Switch2 : Switch  Threshold=1
  Mrs_stDiagnosis : Outport
  Mrs_flgError : Outport  Port=2
  wires:
  Constant6/1 -> Switch2/3
  Relational Operator/1 -> Switch2/2
  Constant5/1 -> Relational Operator/2
  Opm_idxMode_Sim/1 -> Relational Operator/1
  Switch1/1 -> Switch2/1
  dummy_stMainRelais_Sim/1 -> Switch1/3
  Constant2/1 -> Switch1/1
  Constant1/1 -> Switch1/2
  Logical Operator1/1 -> Mrs_flgError/1  "Mrs_flgError"
  G1_DigOut_GetError/1(status) -> Mrs_stDiagnosis/1  "Mrs_stDiagnosis"
  Switch2/1 -> Logical Operator2/1  "Mrs_stMainRelais"
  Logical Operator2/1 -> G1_DigOut_Ctrl/1(state)
  G1_DigOut_Ctrl/1(status) -> Logical Operator1/1

== system Actuators/Actuators_mdl/Str ==
  Opm_idxMode_Sim : Inport
  Stc_stStarter_Sim : Inport  Port=2
  function : TriggerPort  TriggerType=function-call
  Constant1 : Constant  Value=Str_flgStarterOverride
  Constant2 : Constant  Value=Str_stStarterMan
  Constant5 : Constant  Value=Normal
  Constant6 : Constant  Value=0  OutDataTypeStr=boolean
  G1_DigOut_Ctrl : Subsystem  AncestorBlock=ehooks_medc17flex_G1_lib/Library Blocks/Basic_IO/Outputs/G1_DigOut_Ctrl  mask{ChannelName=O_S_RL34}
      mask prompts: ChannelName "Channel name"
      mask init:
      | ehooks_medc17flex_devlib_io_block('mask_init');
      settings: AttributesFormatString=Channel name: '%<ChannelName>'
      mask TypeOptions ChannelName: <empty> | O_S_MRLY | O_S_RL09 | O_S_RL14 | O_S_RL29 | O_S_RL30 | O_S_RL31 | O_S_RL33 | O_S_RL34 | O_S_RL35 | O_S_RL41 | O_S_RL43
      mask Display: image(imread('Output_Digital.jpg'))
  G1_DigOut_GetError : Subsystem  AncestorBlock=ehooks_medc17flex_G1_lib/Library Blocks/Basic_IO/Outputs/G1_DigOut_GetError  mask{ChannelName=O_S_RL34}
      mask prompts: ChannelName "Channel name"
      mask init:
      | ehooks_medc17flex_devlib_io_block('mask_init');
      settings: AttributesFormatString=Channel name: '%<ChannelName>'
      mask TypeOptions ChannelName: <empty> | O_S_MRLY | O_S_RL09 | O_S_RL14 | O_S_RL29 | O_S_RL30 | O_S_RL31 | O_S_RL33 | O_S_RL34 | O_S_RL35 | O_S_RL41 | O_S_RL43
      mask Display: image(imread('Output_Digital_Diagnosis.jpg'))
  Logical Operator1 : Logic  Operator=NOT  AllPortsSameDT=off  OutDataTypeStr=boolean
  Logical Operator2 : Logic  Operator=NOT  AllPortsSameDT=off  OutDataTypeStr=boolean
  Relational Operator : RelationalOperator  Operator===  OutDataTypeStr=boolean
  Switch1 : Switch  Threshold=1
  Switch2 : Switch  Threshold=1
  Str_stDiagnosis : Outport
  Str_flgError : Outport  Port=2
  wires:
  Constant6/1 -> Switch2/3
  Relational Operator/1 -> Switch2/2
  Constant5/1 -> Relational Operator/2
  Opm_idxMode_Sim/1 -> Relational Operator/1
  Switch1/1 -> Switch2/1
  Stc_stStarter_Sim/1 -> Switch1/3
  Constant2/1 -> Switch1/1
  Constant1/1 -> Switch1/2
  Logical Operator1/1 -> Str_flgError/1  "Str_flgError"
  G1_DigOut_GetError/1(status) -> Str_stDiagnosis/1  "Str_stDiagnosis"
  Switch2/1 -> Logical Operator2/1  "Str_stStarter"
  Logical Operator2/1 -> G1_DigOut_Ctrl/1(state)
  G1_DigOut_Ctrl/1(status) -> Logical Operator1/1

== system Actuators/Actuators_mdl/Tvc ==
  Opm_idxMode_Sim : Inport
  dummy_facThrValveReq_Sim : Inport  Port=2
  function : TriggerPort  TriggerType=function-call
  Bus Creator : BusCreator  Inputs=3
  Bus Selector : BusSelector  OutputSignals=Tvc_flgPosError,Tvc_facThrValveReq,Tvc_facThrValve
  Constant1 : Constant  Value=Tvc_flgThrValveReqOverride
  Constant2 : Constant  Value=Tvc_facThrValveReqMan
  Constant3 : Constant  Value=Tvc_facThrValveLimitMax
  Constant4 : Constant  Value=Tvc_facThrValveLimitMin
  Constant5 : Constant  Value=Normal
  Constant6 : Constant  Value=0.0  OutDataTypeStr=single
  Limiter : Subsystem
      mask help: Limiter
      mask Display: image(imread('Limiter.jpg'))
  Logical Operator : Logic  Operator=OR  AllPortsSameDT=off  OutDataTypeStr=boolean
  Logical Operator1 : Logic  Operator=NOT  AllPortsSameDT=off  OutDataTypeStr=boolean
  Relational Operator : RelationalOperator  Operator===  OutDataTypeStr=boolean
  Switch1 : Switch  Threshold=1
  Switch2 : Switch  Threshold=1
  ThrottleValveControl : Subsystem
  ThrottleValveOutput : Subsystem
  ThrottleValvePosition : Subsystem
  Tvc_stDiagnosis : Outport
  Tvc_flgError : Outport  Port=2
  tag scope: Opm_idxMode_global=global
  wires:
  ThrottleValvePosition/1(Tvc_flgPosError) -> Bus Creator/1  "Tvc_flgPosError"
  ThrottleValvePosition/2(Tvc_facThrValve) -> Bus Creator/2  "Tvc_facThrValve"
  Bus Creator/1 -> Bus Selector/1
  Bus Selector/1 -> Logical Operator/1, ThrottleValveOutput/1(Tvc_flgPosError), ThrottleValveControl/1(Tvc_flgPosError)  "<Tvc_flgPosError>"
  Logical Operator1/1 -> Logical Operator/2
  ThrottleValveOutput/1(Tvc_stHBridge) -> Logical Operator1/1
  ThrottleValveControl/1(Tvc_facDutycycle) -> ThrottleValveOutput/2(Tvc_facDutycycle)  "Tvc_facDutycycle"
  Constant3/1 -> Limiter/1(max)
  Constant4/1 -> Limiter/3(min)
  dummy_facThrValveReq_Sim/1 -> Limiter/2(in)
  Constant1/1 -> Switch1/2
  Opm_idxMode_Sim/1 -> [Opm_idxMode_global], Relational Operator/1
  Constant5/1 -> Relational Operator/2
  Relational Operator/1 -> Switch2/2
  Switch1/1 -> Switch2/1
  Switch2/1 -> Bus Creator/3  "Tvc_facThrValveReq"
  Constant6/1 -> Switch2/3
  Logical Operator/1 -> Tvc_flgError/1  "Tvc_flgError"
  Bus Selector/2 -> ThrottleValveControl/2(Tvc_facThrValve)  "<Tvc_facThrValveReq>"
  Bus Selector/3 -> ThrottleValveControl/3(Tvc_facThrValveReq)  "<Tvc_facThrValve>"
  ThrottleValveOutput/2(Tvc_stDiagnosis) -> Tvc_stDiagnosis/1  "Tvc_stDiagnosis"
  Limiter/1(return) -> Switch1/3
  Constant2/1 -> Switch1/1

== system Actuators/Actuators_mdl/Wcs ==
  Opm_idxMode_Sim : Inport
  Ctc_atCool_Sim : Inport  Port=2
  function : TriggerPort  TriggerType=function-call
  Constant1 : Constant  Value=Wcs_flgWaterCoolerOverride
  Constant2 : Constant  Value=Wcs_stWaterCoolerMan
  Constant5 : Constant  Value=Normal
  Constant6 : Constant  Value=0  OutDataTypeStr=boolean
  G1_DigOut_Ctrl : Subsystem  AncestorBlock=ehooks_medc17flex_G1_lib/Library Blocks/Basic_IO/Outputs/G1_DigOut_Ctrl  mask{ChannelName=O_S_RL14}
      mask prompts: ChannelName "Channel name"
      mask init:
      | ehooks_medc17flex_devlib_io_block('mask_init');
      settings: AttributesFormatString=Channel name: '%<ChannelName>'
      mask TypeOptions ChannelName: <empty> | O_S_MRLY | O_S_RL09 | O_S_RL14 | O_S_RL29 | O_S_RL30 | O_S_RL31 | O_S_RL33 | O_S_RL34 | O_S_RL35 | O_S_RL41 | O_S_RL43
      mask Display: image(imread('Output_Digital.jpg'))
  G1_DigOut_GetError : Subsystem  AncestorBlock=ehooks_medc17flex_G1_lib/Library Blocks/Basic_IO/Outputs/G1_DigOut_GetError  mask{ChannelName=O_S_RL14}
      mask prompts: ChannelName "Channel name"
      mask init:
      | ehooks_medc17flex_devlib_io_block('mask_init');
      settings: AttributesFormatString=Channel name: '%<ChannelName>'
      mask TypeOptions ChannelName: <empty> | O_S_MRLY | O_S_RL09 | O_S_RL14 | O_S_RL29 | O_S_RL30 | O_S_RL31 | O_S_RL33 | O_S_RL34 | O_S_RL35 | O_S_RL41 | O_S_RL43
      mask Display: image(imread('Output_Digital_Diagnosis.jpg'))
  Hysteresis_Delta_RSP : Subsystem
      mask help: Hysteresis_Delta_RSP
      mask Display: image(imread('HysteresDeltaR.jpg'))
  Logical Operator1 : Logic  Operator=NOT  AllPortsSameDT=off  OutDataTypeStr=boolean
  Logical Operator2 : Logic  Operator=NOT  AllPortsSameDT=off  OutDataTypeStr=boolean
  Relational Operator : RelationalOperator  Operator===  OutDataTypeStr=boolean
  Switch1 : Switch  Threshold=1
  Switch2 : Switch  Threshold=1
  Wcs_stDiagnosis : Outport
  Wcs_flgError : Outport  Port=2
  wires:
  Constant6/1 -> Switch2/3
  Relational Operator/1 -> Switch2/2
  Constant5/1 -> Relational Operator/2
  Opm_idxMode_Sim/1 -> Relational Operator/1
  Switch1/1 -> Switch2/1
  Ctc_atCool_Sim/1 -> Hysteresis_Delta_RSP/1(in)
  Constant2/1 -> Switch1/1
  Constant1/1 -> Switch1/2
  Logical Operator1/1 -> Wcs_flgError/1  "Wcs_flgError"
  G1_DigOut_GetError/1(status) -> Wcs_stDiagnosis/1  "Wcs_stDiagnosis"
  Switch2/1 -> Logical Operator2/1  "Wcs_stWaterCooler"
  Logical Operator2/1 -> G1_DigOut_Ctrl/1(state)
  G1_DigOut_Ctrl/1(status) -> Logical Operator1/1
  Hysteresis_Delta_RSP/1(return) -> Switch1/3

== system Actuators/Actuators_mdl/Wgc ==
  Opm_idxMode_Sim : Inport
  T2t_facWasteGateRate_Sim : Inport  Port=2
  function : TriggerPort  TriggerType=function-call
  Constant1 : Constant  Value=Wgc_flgWastegateRateOverride
  Constant2 : Constant  Value=Wgc_facWasteGateRateMan
  Constant3 : Constant  Value=10000  OutDataTypeStr=single
  Constant4 : Constant  Value=Wgc_factor
  Constant5 : Constant  Value=Normal
  Constant6 : Constant  Value=0.0  OutDataTypeStr=single
  Constant7 : Constant  Value=Wgc_tiPeriod_C
  Constant9 : Constant  Value=Lo_
  G1_PWM_Output_Ctrl : Subsystem  AncestorBlock=ehooks_medc17flex_G1_lib/Library Blocks/Basic_IO/Outputs/G1_PWM_Output_Ctrl  mask{ChannelName=O_T_RL22}
      mask prompts: ChannelName "Channel name"
      mask init:
      | ehooks_medc17flex_devlib_io_block('mask_init');
      settings: AttributesFormatString=Channel name: '%<ChannelName>'
      mask TypeOptions ChannelName: <empty> | O_T_RL10 | O_T_RL13 | O_T_RL19 | O_T_RL20 | O_T_RL22 | O_T_RL23 | O_T_RL25 | O_T_RL26 | O_T_RL27 | O_T_RL28 | O_T_RL38 | O_T_RL39 | O_T_RL40 | O_T_RL42 | O_T_RL44 | O_T_RL45 | O_T_RL46 | O_T_RL47 | O_T_RL48 | O_T_RL49 | O_T_RL50 | O_T_RH02
      mask Display: image(imread('Output_PWM.jpg'))
  G1_PwmOut_Get_error : Subsystem  AncestorBlock=ehooks_medc17flex_G1_lib/Library Blocks/Basic_IO/Outputs/G1_PwmOut_Get_error  mask{ChannelName=O_T_RL22}
      mask prompts: ChannelName "Channel name"
      mask init:
      | ehooks_medc17flex_devlib_io_block('mask_init');
      settings: AttributesFormatString=Channel name: '%<ChannelName>'
      mask TypeOptions ChannelName: <empty> | O_T_RL10 | O_T_RL13 | O_T_RL19 | O_T_RL20 | O_T_RL22 | O_T_RL23 | O_T_RL25 | O_T_RL26 | O_T_RL27 | O_T_RL28 | O_T_RL38 | O_T_RL39 | O_T_RL40 | O_T_RL42 | O_T_RL44 | O_T_RL45 | O_T_RL46 | O_T_RL47 | O_T_RL48 | O_T_RL49 | O_T_RL50 | O_T_RH02
      mask Display: image(imread('Output_PWM_Diagnosis.jpg'))
  Logical Operator1 : Logic  Operator=NOT  AllPortsSameDT=off  OutDataTypeStr=boolean
  Product1 : Product  OutDataTypeStr=Inherit: Same as first input
  Relational Operator : RelationalOperator  Operator===  OutDataTypeStr=boolean
  Switch1 : Switch  Threshold=1
  Switch2 : Switch  Threshold=1
  Wgc_stDiagnosis : Outport
  Wgc_flgError : Outport  Port=2
  wires:
  Constant6/1 -> Switch2/3
  Relational Operator/1 -> Switch2/2
  Constant5/1 -> Relational Operator/2
  Opm_idxMode_Sim/1 -> Relational Operator/1
  Switch1/1 -> Switch2/1
  T2t_facWasteGateRate_Sim/1 -> Switch1/3
  Constant2/1 -> Switch1/1
  Constant1/1 -> Switch1/2
  Logical Operator1/1 -> Wgc_flgError/1  "Wgc_flgError"
  G1_PwmOut_Get_error/1(status) -> Wgc_stDiagnosis/1  "Wgc_stDiagnosis"
  Switch2/1 -> Product1/1  "Wgc_facWasteGateRate"
  G1_PWM_Output_Ctrl/1(status) -> Logical Operator1/1
  Constant3/1 -> Product1/2
  Product1/1 -> G1_PWM_Output_Ctrl/1(dutycycle)
  Constant7/1 -> G1_PWM_Output_Ctrl/2(period)
  Constant4/1 -> G1_PWM_Output_Ctrl/3(factor)
  Constant9/1 -> G1_PWM_Output_Ctrl/4(level)

== system Actuators/Actuators_mdl/Ais/G1_DigOut_Ctrl ==
  state : Inport
  DTC_DigOut_ctrl : DataTypeConversion  OutDataTypeStr=uint8  RndMeth=Nearest
  DTC_Out1 : DataTypeConversion  OutDataTypeStr=boolean
  FlexECU_DevLib_FcnAPI_Wrapper_SFcn : S-Function  FunctionName=ehooks_medc17flex_devlib_basic_io_fcncall  Parameters=NoInputPorts, NoOutputPorts, InputPortDataTypes, OutputPortDataTypes, CFunctionArgTypes, CFunctionName, ChannelName  EnableBusSupport=off  mask{NoInputPorts=1, NoOutputPorts=1, InputPortDataTypes=uint8, OutputPortDataTypes=uint8, CFunctionArgTypes=ret,val, CFunctionName=DevLib_Dio_Set, ChannelName=O_S_RL30}
      mask prompts: NoInputPorts "Number of input ports"; NoOutputPorts "Number of output ports"; InputPortDataTypes "Input port data types"; OutputPortDataTypes "Output port data types"; CFunctionArgTypes "C function argument types"; CFunctionName "C function name"; ChannelName "Channel (pin) name"
      mask Display: disp('EHOOKS FlexECU\nDevLib Wrapper\nS-Function')
  status : Outport
  wires:
  DTC_Out1/1 -> status/1
  FlexECU_DevLib_FcnAPI_Wrapper_SFcn/1 -> DTC_Out1/1
  state/1 -> DTC_DigOut_ctrl/1
  DTC_DigOut_ctrl/1 -> FlexECU_DevLib_FcnAPI_Wrapper_SFcn/1

== system Actuators/Actuators_mdl/Ais/G1_DigOut_GetError ==
  DTC_DigOut_GetError : DataTypeConversion  OutDataTypeStr=single
  FlexECU_DevLib_FcnAPI_Wrapper_SFcn : S-Function  FunctionName=ehooks_medc17flex_devlib_basic_io_fcncall  Parameters=NoInputPorts, NoOutputPorts, InputPortDataTypes, OutputPortDataTypes, CFunctionArgTypes, CFunctionName, ChannelName  EnableBusSupport=off  mask{NoInputPorts=0, NoOutputPorts=1, InputPortDataTypes=, OutputPortDataTypes=uint8, CFunctionArgTypes=ret, CFunctionName=DevLib_DioSet_GetError, ChannelName=O_S_RL30}
      mask prompts: NoInputPorts "Number of input ports"; NoOutputPorts "Number of output ports"; InputPortDataTypes "Input port data types"; OutputPortDataTypes "Output port data types"; CFunctionArgTypes "C function argument types"; CFunctionName "C function name"; ChannelName "Channel (pin) name"
      mask Display: disp('EHOOKS FlexECU\nDevLib Wrapper\nS-Function')
  status : Outport
  wires:
  FlexECU_DevLib_FcnAPI_Wrapper_SFcn/1 -> DTC_DigOut_GetError/1
  DTC_DigOut_GetError/1 -> status/1
